simulink model "week1prob5"  (R2020b)
settings: Solver=VariableStepAuto  StartTime=0.0  StopTime=10.0  RelTol=1e-3
model workspace (MAT data in the model file):
  C = Simulink.Parameter
  C.Value = 1e-05
  C.DataType = 'auto'
  C.Dimensions = [1 1]
  R = Simulink.Parameter
  R.Value = 10
  R.DataType = 'auto'
  R.Dimensions = [1 1]
settings Model: Creator=lalit  LastModifiedBy=lalit

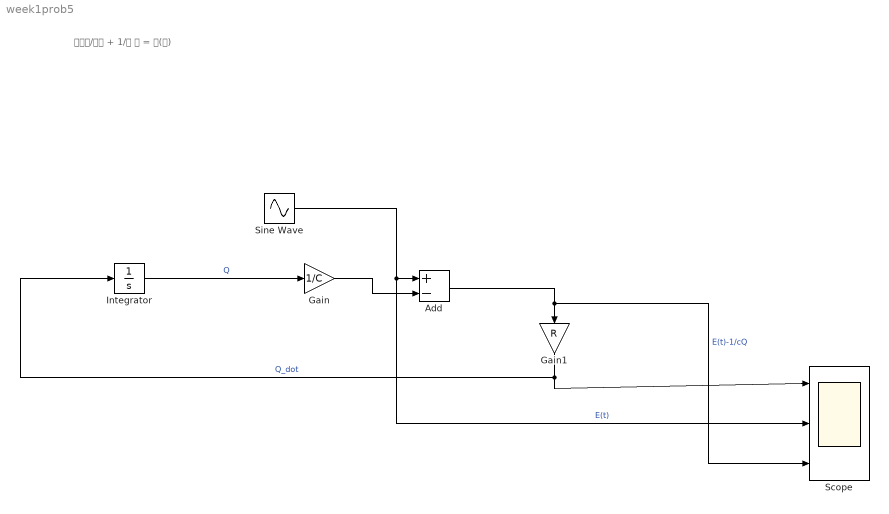
== system week1prob5 ==
  note: 𝑅𝑑𝑄/𝑑𝑡 + 1/𝐶 𝑄 = 𝐸(𝑡)
  Add : Sum  Inputs=+-
  Gain : Gain  Gain=1/C
  Gain1 : Gain  Gain=R
  Integrator : Integrator
  Scope : Scope  NumInputPorts=3
  Sine Wave : Sin  Amplitude=5  Frequency=10  SampleTime=0
  wires:
  Integrator/1 -> Gain/1  "Q"
  Gain/1 -> Add/2
  Sine Wave/1 -> Scope/2, Add/1  "E(t)"
  Add/1 -> Scope/3, Gain1/1  "E(t)-1/cQ"
  Gain1/1 -> Integrator/1, Scope/1  "Q_dot"
